simulink model "green_joint_current_loop_model"  (R2023b)
settings: Solver=FixedStepDiscrete  StartTime=0.0  StopTime=0.001  FixedStep=5e-05  RelTol=1e-3
values from neighbouring files (symbols this model uses):
  CurDKi = 23812.2981754    [green_joint_current_loop_interface.sldd]
  CurDKp = 1.52320723148    [green_joint_current_loop_interface.sldd]
  CurQKi = 23812.2981754    [green_joint_current_loop_interface.sldd]
  CurQKp = 1.52320723148    [green_joint_current_loop_interface.sldd]
  PiCorrectionGain = 400.0    [green_joint_current_loop_interface.sldd]
  VoltageEpsilon = 0.001    [green_joint_current_loop_interface.sldd]
  VoltageLimitRatio = 0.577    [green_joint_current_loop_interface.sldd]
  VoltageModulationRatio = 0.9    [green_joint_current_loop_interface.sldd]
settings Model: DataDictionary=green_joint_current_loop_interface.sldd  Creator=user  LastModifiedBy=user
settings OptimizationCC: EnhancedBackFolding=on  PassReuseOutputArgsAs=Individual arguments  OptimizeBlockOrder=speed  DifferentSizesBufferReuse=on  OptimizationCustomize=off  EfficientTunableParamExpr=on
settings DebuggingCC: ParameterPrecisionLossMsg=none  ParameterTunabilityLossMsg=error
settings HardwareCC: ProdBitPerPointer=32  ProdBitPerSizeT=32  ProdBitPerPtrDiffT=32  ProdLargestAtomicInteger=Long  ProdLargestAtomicFloat=Double  ProdWordSize=32  ProdHWDeviceType=ARM Compatible->ARM Cortex  TargetLargestAtomicInteger=Long  TargetLargestAtomicFloat=Double  TargetIntDivRoundTo=Zero  TargetEndianess=LittleEndian  TargetHWDeviceType=ARM Compatible->ARM Cortex  ProdEqTarget=off
settings SFSimCC: MATLABDynamicMemAlloc=off
settings RTWCC: Description=Embedded Coder  SystemTargetFile=ert.tlc  GenCodeOnly=on  TemplateMakefile=ert_default_tmf  GenerateReport=on
settings CodeAppCC: ForceParamTrailComments=on  IgnoreCustomStorageClasses=off  OperatorAnnotations=on  SimulinkDataObjDesc=on  SFDataObjDesc=on  InsertBlockDesc=on
settings ERTTargetCC: TargetLangStandard=C99 (ISO)  CodeInterfacePackaging=Reusable function  ERTCustomFileTemplate=example_file_process.tlc

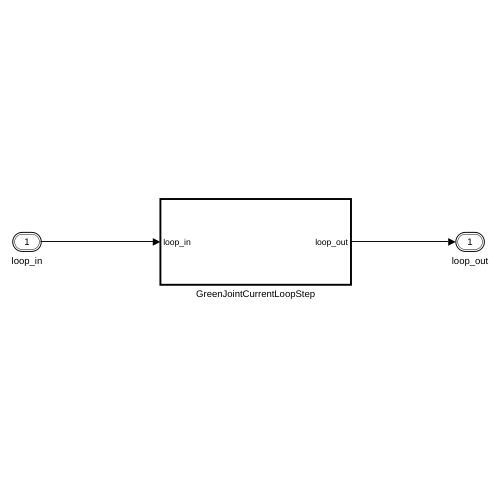
[thumbnail: Simulink's stored preview of the top-level diagram]
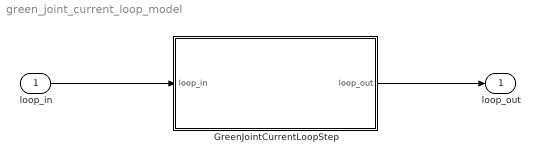
== system green_joint_current_loop_model ==
  loop_in : Inport  OutDataTypeStr=Bus: green_joint_current_loop_input_t  BusOutputAsStruct=on
  GreenJointCurrentLoopStep : Subsystem  TreatAsAtomicUnit=on  RTWFcnName=GreenJointCurrentLoopStep  RTWFileName=GreenJointCurrentLoopStep
      settings: RTWFcnNameOpts=User specified  RTWFileNameOpts=User specified
  loop_out : Outport  OutDataTypeStr=Bus: green_joint_current_loop_output_t
  wires:
  loop_in/1 -> GreenJointCurrentLoopStep/1(loop_in)
  GreenJointCurrentLoopStep/1(loop_out) -> loop_out/1

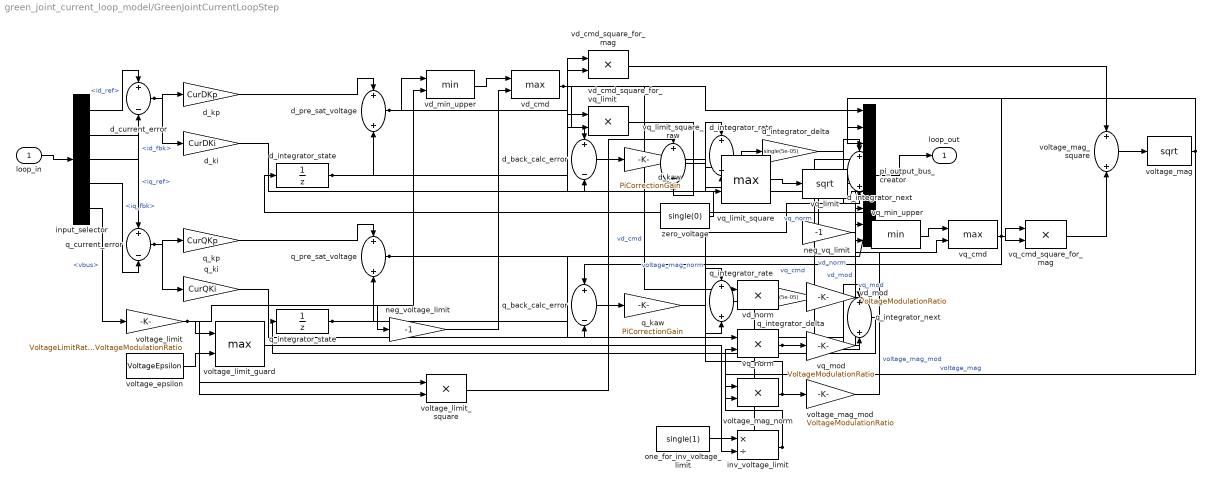
== system green_joint_current_loop_model/GreenJointCurrentLoopStep ==
  loop_in : Inport  OutDataTypeStr=Bus: green_joint_current_loop_input_t  BusOutputAsStruct=on
  d_back_calc_error : Sum  Inputs=+-  OutDataTypeStr=T_GJVoltage  AccumDataTypeStr=T_GJVoltage
  d_current_error : Sum  Inputs=+-  OutDataTypeStr=T_GJCurrent  AccumDataTypeStr=T_GJCurrent
  d_integrator_delta : Gain  Gain=single(5e-05)  ParamDataTypeStr=T_GJFloat  OutDataTypeStr=T_GJVoltage
  d_integrator_next : Sum  OutDataTypeStr=T_GJVoltage  AccumDataTypeStr=T_GJVoltage
  d_integrator_rate : Sum  OutDataTypeStr=T_GJVoltage  AccumDataTypeStr=T_GJVoltage
  d_integrator_state : UnitDelay  InitialCondition=single(0)  SampleTime=5e-05  HasFrameUpgradeWarning=on
  d_kaw : Gain  Gain=PiCorrectionGain  ParamDataTypeStr=T_GJFloat  OutDataTypeStr=T_GJVoltage
  d_ki : Gain  Gain=CurDKi  ParamDataTypeStr=T_GJFloat  OutDataTypeStr=T_GJVoltage
  d_kp : Gain  Gain=CurDKp  ParamDataTypeStr=T_GJFloat  OutDataTypeStr=T_GJVoltage
  d_pre_sat_voltage : Sum  OutDataTypeStr=T_GJVoltage  AccumDataTypeStr=T_GJVoltage
  input_selector : BusSelector  OutputSignals=id_ref,iq_ref,id_fbk,iq_fbk,vbus
  inv_voltage_limit : Product  Inputs=*/  OutDataTypeStr=T_GJFloat
  neg_voltage_limit : Gain  Gain=-1  ParamDataTypeStr=T_GJFloat  OutDataTypeStr=T_GJVoltage
  neg_vq_limit : Gain  Gain=-1  ParamDataTypeStr=T_GJFloat  OutDataTypeStr=T_GJVoltage
  one_for_inv_voltage_limit : Constant  Value=single(1)  OutDataTypeStr=T_GJFloat  SampleTime=-1
  pi_output_bus_creator : BusCreator  Inputs=9  OutDataTypeStr=Bus: green_joint_current_loop_output_t  NonVirtualBus=on
  q_back_calc_error : Sum  Inputs=+-  OutDataTypeStr=T_GJVoltage  AccumDataTypeStr=T_GJVoltage
  q_current_error : Sum  Inputs=+-  OutDataTypeStr=T_GJCurrent  AccumDataTypeStr=T_GJCurrent
  q_integrator_delta : Gain  Gain=single(5e-05)  ParamDataTypeStr=T_GJFloat  OutDataTypeStr=T_GJVoltage
  q_integrator_next : Sum  OutDataTypeStr=T_GJVoltage  AccumDataTypeStr=T_GJVoltage
  q_integrator_rate : Sum  OutDataTypeStr=T_GJVoltage  AccumDataTypeStr=T_GJVoltage
  q_integrator_state : UnitDelay  InitialCondition=single(0)  SampleTime=5e-05  HasFrameUpgradeWarning=on
  q_kaw : Gain  Gain=PiCorrectionGain  ParamDataTypeStr=T_GJFloat  OutDataTypeStr=T_GJVoltage
  q_ki : Gain  Gain=CurQKi  ParamDataTypeStr=T_GJFloat  OutDataTypeStr=T_GJVoltage
  q_kp : Gain  Gain=CurQKp  ParamDataTypeStr=T_GJFloat  OutDataTypeStr=T_GJVoltage
  q_pre_sat_voltage : Sum  OutDataTypeStr=T_GJVoltage  AccumDataTypeStr=T_GJVoltage
  vd_cmd : MinMax  Function=max  Inputs=2
  vd_cmd_square_for_mag : Product  Inputs=**  OutDataTypeStr=T_GJVoltage
  vd_cmd_square_for_vq_limit : Product  Inputs=**  OutDataTypeStr=T_GJVoltage
  vd_min_upper : MinMax  Inputs=2
  vd_mod : Gain  Gain=VoltageModulationRatio  ParamDataTypeStr=T_GJFloat  OutDataTypeStr=T_GJVoltageNorm
  vd_norm : Product  Inputs=**  OutDataTypeStr=T_GJVoltageNorm
  voltage_epsilon : Constant  Value=VoltageEpsilon  OutDataTypeStr=T_GJVoltage  SampleTime=-1
  voltage_limit : Gain  Gain=VoltageLimitRatio * VoltageModulationRatio  ParamDataTypeStr=T_GJFloat  OutDataTypeStr=T_GJVoltage
  voltage_limit_guard : MinMax  Function=max  Inputs=2
  voltage_limit_square : Product  Inputs=**  OutDataTypeStr=T_GJVoltage
  voltage_mag : Math  Operator=sqrt  OutDataTypeStr=T_GJVoltage
  voltage_mag_mod : Gain  Gain=VoltageModulationRatio  ParamDataTypeStr=T_GJFloat  OutDataTypeStr=T_GJVoltageNorm
  voltage_mag_norm : Product  Inputs=**  OutDataTypeStr=T_GJVoltageNorm
  voltage_mag_square : Sum  OutDataTypeStr=T_GJVoltage  AccumDataTypeStr=T_GJVoltage
  vq_cmd : MinMax  Function=max  Inputs=2
  vq_cmd_square_for_mag : Product  Inputs=**  OutDataTypeStr=T_GJVoltage
  vq_limit : Math  Operator=sqrt  OutDataTypeStr=T_GJVoltage
  vq_limit_square : MinMax  Function=max  Inputs=2
  vq_limit_square_raw : Sum  Inputs=+-  OutDataTypeStr=T_GJVoltage  AccumDataTypeStr=T_GJVoltage
  vq_min_upper : MinMax  Inputs=2
  vq_mod : Gain  Gain=VoltageModulationRatio  ParamDataTypeStr=T_GJFloat  OutDataTypeStr=T_GJVoltageNorm
  vq_norm : Product  Inputs=**  OutDataTypeStr=T_GJVoltageNorm
  zero_voltage : Constant  Value=single(0)  OutDataTypeStr=T_GJVoltage  SampleTime=-1
  loop_out : Outport  OutDataTypeStr=Bus: green_joint_current_loop_output_t
  wires:
  loop_in/1 -> input_selector/1
  input_selector/5 -> voltage_limit/1  "<vbus>"
  voltage_limit/1 -> voltage_limit_guard/1, neg_voltage_limit/1, vd_min_upper/2, voltage_limit_square/1, voltage_limit_square/2
  voltage_epsilon/1 -> voltage_limit_guard/2
  input_selector/1 -> d_current_error/1  "<id_ref>"
  input_selector/3 -> d_current_error/2  "<id_fbk>"
  d_current_error/1 -> d_kp/1, d_ki/1
  d_kp/1 -> d_pre_sat_voltage/1
  d_integrator_state/1 -> d_pre_sat_voltage/2, d_integrator_next/1
  d_ki/1 -> d_integrator_rate/1
  d_back_calc_error/1 -> d_kaw/1
  d_kaw/1 -> d_integrator_rate/2
  d_integrator_rate/1 -> d_integrator_delta/1
  d_integrator_delta/1 -> d_integrator_next/2
  d_integrator_next/1 -> d_integrator_state/1
  input_selector/2 -> q_current_error/1  "<iq_ref>"
  input_selector/4 -> q_current_error/2  "<iq_fbk>"
  q_current_error/1 -> q_kp/1, q_ki/1
  q_kp/1 -> q_pre_sat_voltage/1
  q_integrator_state/1 -> q_pre_sat_voltage/2, q_integrator_next/1
  q_ki/1 -> q_integrator_rate/1
  q_back_calc_error/1 -> q_kaw/1
  q_kaw/1 -> q_integrator_rate/2
  q_integrator_rate/1 -> q_integrator_delta/1
  q_integrator_delta/1 -> q_integrator_next/2
  q_integrator_next/1 -> q_integrator_state/1
  d_pre_sat_voltage/1 -> vd_min_upper/1, d_back_calc_error/2
  vd_min_upper/1 -> vd_cmd/1
  neg_voltage_limit/1 -> vd_cmd/2
  vd_cmd/1 -> vd_cmd_square_for_vq_limit/1, vd_cmd_square_for_vq_limit/2, vd_cmd_square_for_mag/1, vd_cmd_square_for_mag/2, d_back_calc_error/1, vd_norm/1, pi_output_bus_creator/1  "vd_cmd"
  voltage_limit_square/1 -> vq_limit_square_raw/1
  vd_cmd_square_for_vq_limit/1 -> vq_limit_square_raw/2
  vq_limit_square_raw/1 -> vq_limit_square/1
  zero_voltage/1 -> vq_limit_square/2
  vq_limit_square/1 -> vq_limit/1
  vq_limit/1 -> neg_vq_limit/1, vq_min_upper/2
  q_pre_sat_voltage/1 -> vq_min_upper/1, q_back_calc_error/2
  vq_min_upper/1 -> vq_cmd/1
  neg_vq_limit/1 -> vq_cmd/2
  vq_cmd/1 -> vq_cmd_square_for_mag/1, vq_cmd_square_for_mag/2, q_back_calc_error/1, vq_norm/1, pi_output_bus_creator/2  "vq_cmd"
  vd_cmd_square_for_mag/1 -> voltage_mag_square/1
  vq_cmd_square_for_mag/1 -> voltage_mag_square/2
  voltage_mag_square/1 -> voltage_mag/1
  one_for_inv_voltage_limit/1 -> inv_voltage_limit/1
  voltage_limit_guard/1 -> inv_voltage_limit/2
  inv_voltage_limit/1 -> vd_norm/2, vq_norm/2, voltage_mag_norm/2
  voltage_mag/1 -> voltage_mag_norm/1, pi_output_bus_creator/3  "voltage_mag"
  vd_norm/1 -> vd_mod/1, pi_output_bus_creator/4  "vd_norm"
  vq_norm/1 -> vq_mod/1, pi_output_bus_creator/5  "vq_norm"
  voltage_mag_norm/1 -> voltage_mag_mod/1, pi_output_bus_creator/6  "voltage_mag_norm"
  vd_mod/1 -> pi_output_bus_creator/7  "vd_mod"
  vq_mod/1 -> pi_output_bus_creator/8  "vq_mod"
  voltage_mag_mod/1 -> pi_output_bus_creator/9  "voltage_mag_mod"
  pi_output_bus_creator/1 -> loop_out/1
